simulink model "SIL_DCMotor"  (R2022b)
settings: Solver=VariableStepAuto  StartTime=0.0  StopTime=inf
values from neighbouring files (symbols this model uses):
  b = 0.1    [SIL_DCMotor_Parameter.m]
  J = 0.01    [SIL_DCMotor_Parameter.m]
  Kd_1 = 0.1    [SIL_DCMotor_Parameter.m]
  Kd_2 = 0.1    [SIL_DCMotor_Parameter.m]
  Ke = 0.367    [SIL_DCMotor_Parameter.m]
  Ki_1 = 0.1    [SIL_DCMotor_Parameter.m]
  Ki_2 = 0.75    [SIL_DCMotor_Parameter.m]
  Kp_1 = 0.5    [SIL_DCMotor_Parameter.m]
  Kp_2 = 7.5    [SIL_DCMotor_Parameter.m]
  Kt = 0.367    [SIL_DCMotor_Parameter.m]
  L = 0.5    [SIL_DCMotor_Parameter.m]
  R = 0.1    [SIL_DCMotor_Parameter.m]
  T_L = 0    [SIL_DCMotor_Parameter.m]
  T_sil = 1    [SIL_DCMotor_Parameter.m]
undefined symbols (not defined in the file or in its folder): LF
libraries: fl_lib x5, nesl_utility x4, ee_lib x3, instrumentseriallib x3, slpidlib x2, etargetslib x1
settings Model: Creator=Bramantio  LastModifiedBy=Bramantio

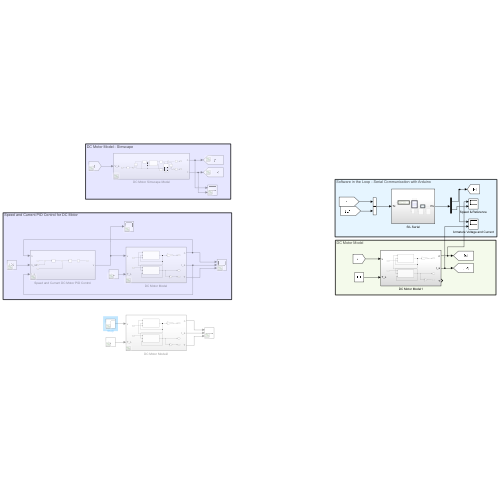
[thumbnail: Simulink's stored preview of the top-level diagram]
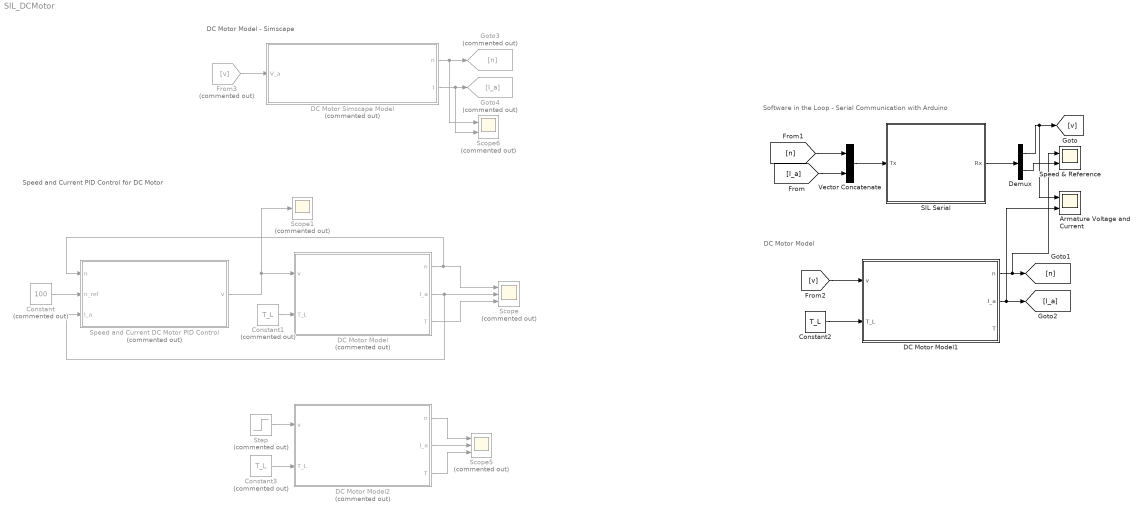
== system SIL_DCMotor ==
  note: DC Motor Model - Simscape
  note: DC Motor Model
  note: Speed and Current PID Control for DC Motor
  note: Software in the Loop - Serial Communication with Arduino
  Armature Voltage and Current : Scope  NumInputPorts=2
  Constant : Constant  Commented=on  Value=100
  Constant1 : Constant  Commented=on  Value=T_L
  Constant2 : Constant  Value=T_L
  Constant3 : Constant  Commented=on  Value=T_L
  DC Motor Model : Subsystem  Commented=on
  DC Motor Model1 : Subsystem
  DC Motor Model2 : Subsystem  Commented=on
  DC Motor Simscape Model : Subsystem  Commented=on
  Demux : Demux  Outputs=2
  From3 : From  Commented=on  GotoTag=v
  Goto3 : Goto  Commented=on  GotoTag=n
  Goto4 : Goto  Commented=on  GotoTag=I_a
  SIL Serial : Subsystem
  Scope : Scope  Commented=on  NumInputPorts=3
  Scope1 : Scope  Commented=on
  Scope5 : Scope  Commented=on  NumInputPorts=3
  Scope6 : Scope  Commented=on  NumInputPorts=2
  Speed & Reference : Scope  NumInputPorts=2
  Speed and Current DC Motor PID Control : Subsystem  Commented=on
  Step : Step  Commented=on  Time=5  After=12  SampleTime=0
  Vector Concatenate : Concatenate
  wires:
  SIL Serial/1(Rx) -> Demux/1
  Demux/2 -> Speed & Reference/2
  [n] -> Vector Concatenate/1
  Demux/1 -> Armature Voltage and Current/1, [v]
  [I_a] -> Vector Concatenate/2
  Vector Concatenate/1 -> SIL Serial/1(Tx)
  DC Motor Model/2(I_a) -> Scope/2, Speed and Current DC Motor PID Control/3(I_a)
  Constant1/1 -> DC Motor Model/2(T_L)
  Constant/1 -> Speed and Current DC Motor PID Control/2(n_ref)
  Speed and Current DC Motor PID Control/1(v) -> Scope1/1, DC Motor Model/1(v)
  DC Motor Model/3(T) -> Scope/3
  DC Motor Model/1(n) -> Scope/1, Speed and Current DC Motor PID Control/1(n)
  Constant2/1 -> DC Motor Model1/2(T_L)
  [v] -> DC Motor Model1/1(v)
  DC Motor Model1/2(I_a) -> Armature Voltage and Current/2, [I_a]
  Constant3/1 -> DC Motor Model2/2(T_L)
  Step/1 -> DC Motor Model2/1(v)
  DC Motor Model2/2(I_a) -> Scope5/2
  DC Motor Model2/1(n) -> Scope5/1
  DC Motor Model2/3(T) -> Scope5/3
  DC Motor Simscape Model/1(n) -> Scope6/1, Goto3/1
  From3/1 -> DC Motor Simscape Model/1(V_a)
  DC Motor Simscape Model/2(I) -> Scope6/2, Goto4/1
  DC Motor Model1/1(n) -> Speed & Reference/1, [n]

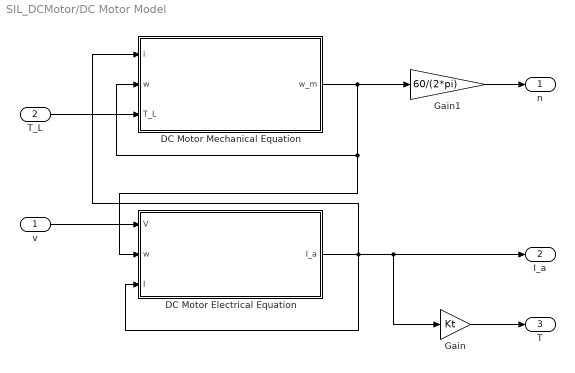
== system SIL_DCMotor/DC Motor Model ==
  v : Inport
  T_L : Inport  Port=2
  DC Motor Electrical Equation : Subsystem
  DC Motor Mechanical Equation : Subsystem
  Gain : Gain  Gain=Kt
  Gain1 : Gain  Gain=60/(2*pi)
  n : Outport
  I_a : Outport  Port=2
  T : Outport  Port=3
  wires:
  DC Motor Mechanical Equation/1(w_m) -> Gain1/1, DC Motor Electrical Equation/2(w), DC Motor Mechanical Equation/2(w)
  v/1 -> DC Motor Electrical Equation/1(V)
  Gain1/1 -> n/1
  DC Motor Electrical Equation/1(I_a) -> DC Motor Mechanical Equation/1(i), Gain/1, I_a/1, DC Motor Electrical Equation/3(I)
  Gain/1 -> T/1
  T_L/1 -> DC Motor Mechanical Equation/3(T_L)

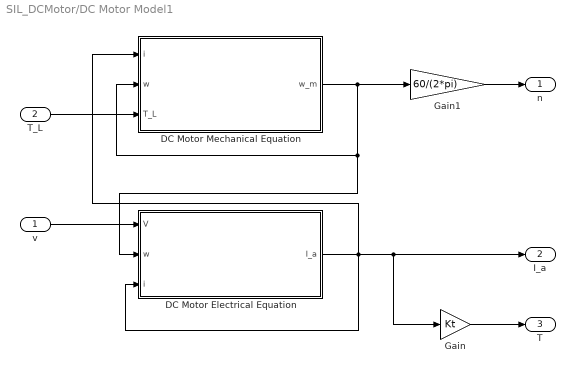
== system SIL_DCMotor/DC Motor Model1 ==
  v : Inport
  T_L : Inport  Port=2
  DC Motor Electrical Equation : Subsystem
  DC Motor Mechanical Equation : Subsystem
  Gain : Gain  Gain=Kt
  Gain1 : Gain  Gain=60/(2*pi)
  n : Outport
  I_a : Outport  Port=2
  T : Outport  Port=3
  wires:
  DC Motor Mechanical Equation/1(w_m) -> Gain1/1, DC Motor Electrical Equation/2(w), DC Motor Mechanical Equation/2(w)
  v/1 -> DC Motor Electrical Equation/1(V)
  Gain1/1 -> n/1
  DC Motor Electrical Equation/1(I_a) -> DC Motor Mechanical Equation/1(i), Gain/1, I_a/1, DC Motor Electrical Equation/3(i)
  Gain/1 -> T/1
  T_L/1 -> DC Motor Mechanical Equation/3(T_L)

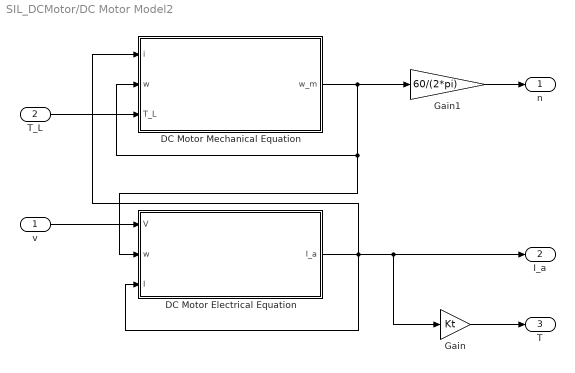
== system SIL_DCMotor/DC Motor Model2 ==
  v : Inport
  T_L : Inport  Port=2
  DC Motor Electrical Equation : Subsystem
  DC Motor Mechanical Equation : Subsystem
  Gain : Gain  Gain=Kt
  Gain1 : Gain  Gain=60/(2*pi)
  n : Outport
  I_a : Outport  Port=2
  T : Outport  Port=3
  wires:
  DC Motor Mechanical Equation/1(w_m) -> Gain1/1, DC Motor Electrical Equation/2(w), DC Motor Mechanical Equation/2(w)
  v/1 -> DC Motor Electrical Equation/1(V)
  Gain1/1 -> n/1
  DC Motor Electrical Equation/1(I_a) -> DC Motor Mechanical Equation/1(i), Gain/1, I_a/1, DC Motor Electrical Equation/3(I)
  Gain/1 -> T/1
  T_L/1 -> DC Motor Mechanical Equation/3(T_L)

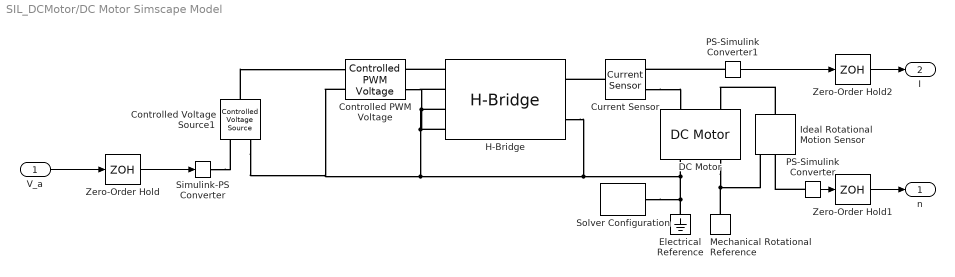
== system SIL_DCMotor/DC Motor Simscape Model ==
  V_a : Inport
  Controlled PWM Voltage : ee_lib/Integrated Circuits/Controlled PWM Voltage  F=4000 Hz  TD=0 s  pulse_width_offset=0 s  pulse_min=0 s  pwm_or_av=ee.enum.pwm_or_av.averaged  event_type=ee.enum.ic.event.asynchronous  sample_time=1e-6 s  Vmin=0 V  Vmax=5 V  Vm=5 V  u_min=0  u_max=1
  Controlled Voltage Source1 : fl_lib/Electrical/Electrical Sources/Controlled Voltage Source
  Current Sensor : fl_lib/Electrical/Electrical Sensors/Current Sensor
  DC Motor : ee_lib/Electromechanical/Brushed Motors/DC Motor  field_option=ee.enum.field_option.pm  Rf=100 Ohm  Lf=1 H  Laf=0.15 H  If0=0 A  parameterization=ee.enum.dcparam_option.circuit_param  Ra=R Ohm  La=L H  emf_or_torque=ee.enum.emf_or_torque.ki  Kv=Kt V/rpm  Ki=Ke N*m/A  T_stall=0.24e-3 N*m  w_max=4000 rpm  w_rated=2500 rpm  P_rated=10 W  V_rated=12 V  lam_param=ee.enum.lam_param.damping  i_noload=0 A  V_i_noload=1.5 V  J=J kg*m^2  lam=b N*m*s/rad  speed0=0 rpm  enable_fault_armature=simscape.enum.onoff.off  rev_faulted=1 / 3  G_faulted_armature=1e-5 S  fault_trigger_armature=ee.enum.faults.faultTrigger.temporal  t_fault_armature=1 s  max_permissible_current_armature=inf A  t_fail_on_current_armature=1 s  enable_fault_field=simscape.enum.onoff.off  G_faulted_field=1e-5 S  fault_trigger_field=ee.enum.faults.faultTrigger.temporal  t_fault_field=1 s  max_permissible_current_field=inf A  t_fail_on_current_field=1 s  fault_action=simscape.enum.assert.action.none  alpha=3.93e-3 1/K  Tmeas=25 degC  thermal_mass=100 J/K  initial_temperature=25 degC
  Electrical Reference : fl_lib/Electrical/Electrical Elements/Electrical Reference
  H-Bridge : ee_lib/Semiconductors & Converters/Converters/H-Bridge  supply_ports=ee.enum.supply_ports.hidesupply  pwm_or_av=ee.enum.pwm_or_av.averaged  regenerative_braking_mode=ee.enum.converters.regenerative_braking_mode.depends_on_rev  discontinuous=ee.enum.current_profile.continuous  freewheeling_mode=ee.enum.converters.freewheeling_mode.one_switch_one_diode  Rload=10 Ohm  Lload=1e-5 H  F=10 kHz  Venable=2.5 V  Vmax=5.0 V  Vreverse=2.5 V  Vbrake=2.5 V  Vm=12 V  Ron=0.1 Ohm  Don=0.05 Ohm  Goff=1e-6 S  Tmeas=298.15 K  Ron2=0.1 Ohm  Don2=0.05 Ohm  Tmeas2=398.15 K  thermal_mass=100 J/K  initial_temperature=298.15 K
  Ideal Rotational Motion Sensor : fl_lib/Mechanical/Mechanical Sensors/Ideal Rotational Motion Sensor  reference=foundation.enum.MeasurementReference.difference  acceleration_port=false  velocity_port=true  position_port=true  wrap_angle=false  offset=0 rad
  Mechanical Rotational Reference : fl_lib/Mechanical/Rotational Elements/Mechanical Rotational Reference
  PS-Simulink Converter : nesl_utility/PS-Simulink Converter  PhysicalDomain=network_engine_domain  SubClassName=ps_output  LeftPortType=input  RightPortType=output  PseudoPeriodic=off  Frequencies=[]  VectorFormat=inherit  Unit=rpm  AffineConversion=off
  PS-Simulink Converter1 : nesl_utility/PS-Simulink Converter  PhysicalDomain=network_engine_domain  SubClassName=ps_output  LeftPortType=input  RightPortType=output  PseudoPeriodic=off  Frequencies=[]  VectorFormat=inherit  Unit=A  AffineConversion=off
  Simulink-PS Converter : nesl_utility/Simulink-PS Converter  PhysicalDomain=network_engine_domain  SubClassName=ps_input  LeftPortType=input  RightPortType=output  PseudoPeriodic=off  Frequencies=[]  NoiseDistribution=none  NoiseParameters=[]  Unit=1  AffineConversion=off  FilteringAndDerivatives=provide  SimscapeFilterOrder=1  InputFilterTimeConstant=0.001  UdotUserProvided=0
  Solver Configuration : nesl_utility/Solver Configuration  PhysicalDomain=network_engine_domain  SubClassName=solver  LeftPortType=input  RightPortType=generic  Tones=[]  Harmonics=[]  SimulateNoise=off  Profile=off  UseLocalSampling=off  EnableSwitchedLinearOptims=on  FrequencyDomain=off  UseCCode=off  RelTol=0.001  AbsTol=0.001  MinStep=1e-09  ToWorkspace=off  RevertToSquareIcSolve=off  NumHomotopyIterations=100  PhasorMode=off  PhasorModeNumHarmonics=1  ConsistencySolver=NEWTON_XTOL_AFTER_FTOL  IndexReductionMethod=DerivativeReplacement  DoDC=off  ResidualTolerance=1e-09  ConsistencyTolSource=GLOBAL  ConsistencyAbsTol=0.001  ConsistencyRelTol=0.001  ConsistencyTolFactor=0.001  UseLocalSolver=off  LocalSolverChoice=NE_BACKWARD_EULER_ADVANCER  ResolveIndetEquations=on  FunctionEvalNumThread=1  LocalSolverSampleTime=0.001  DoFixedCost=off  MaxNonlinIter=3  MaxModeIter=2  ComputeImpulses=off  ImpulseIterations=2  LinearAlgebra=auto  LinearAlgebraNumThread=0  EquationFormulation=NE_TIME_EF  DelaysMemoryBudget=1024  AutomaticFiltering=on  FilteringTimeConstant=0.001  PartitionStorageMethod=AS_NEEDED  PartitionMemoryBudget=1024  PartitionMethod=ROBUST
  Zero-Order Hold : ZeroOrderHold  SampleTime=T_sil
  Zero-Order Hold1 : ZeroOrderHold  SampleTime=T_sil
  Zero-Order Hold2 : ZeroOrderHold  SampleTime=T_sil
  n : Outport
  I : Outport  Port=2
  wires:
  PS-Simulink Converter1/1 -> Zero-Order Hold2/1
  V_a/1 -> Zero-Order Hold/1
  Zero-Order Hold/1 -> Simulink-PS Converter/1
  PS-Simulink Converter/1 -> Zero-Order Hold1/1
  Zero-Order Hold1/1 -> n/1
  Zero-Order Hold2/1 -> I/1
  connections:
  Current Sensor/LConn1 -- H-Bridge/RConn1
  Electrical Reference/LConn1 -- Solver Configuration/RConn1 -- H-Bridge/RConn2 -- Controlled Voltage Source1/RConn2 -- Controlled PWM Voltage/LConn2 -- Controlled PWM Voltage/RConn2 -- H-Bridge/LConn2 -- H-Bridge/LConn3 -- H-Bridge/LConn4 -- DC Motor/RConn1
  Controlled Voltage Source1/LConn1 -- Controlled PWM Voltage/LConn1
  Current Sensor/RConn2 -- DC Motor/LConn1
  H-Bridge/LConn1 -- Controlled PWM Voltage/RConn1
  PS-Simulink Converter1/LConn1 -- Current Sensor/RConn1
  Mechanical Rotational Reference/LConn1 -- DC Motor/RConn2 -- Ideal Rotational Motion Sensor/RConn1
  PS-Simulink Converter/LConn1 -- Ideal Rotational Motion Sensor/RConn2
  Ideal Rotational Motion Sensor/LConn1 -- DC Motor/LConn2
  Simulink-PS Converter/RConn1 -- Controlled Voltage Source1/RConn1

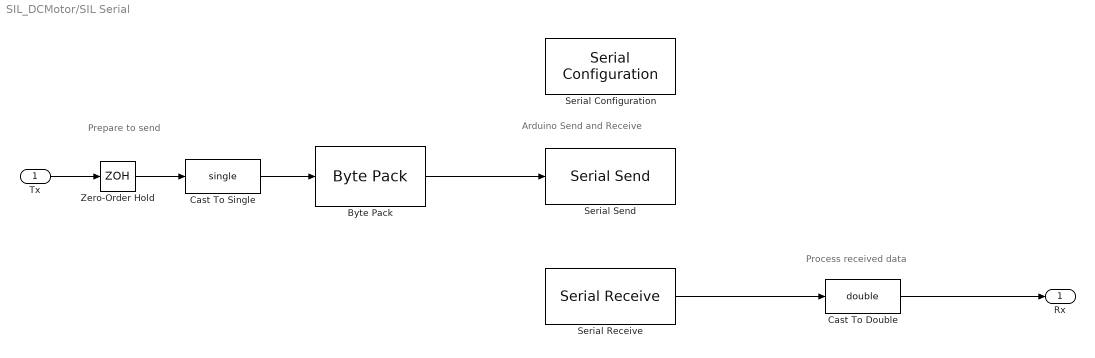
== system SIL_DCMotor/SIL Serial ==
  note: Prepare to send
  note: Arduino Send and Receive
  note: Process received data
  Tx : Inport
  Byte Pack : etargetslib/Byte Pack  datatypes={'single'}  byteAlign=4
  Cast To Double : DataTypeConversion  OutDataTypeStr=double  SaturateOnIntegerOverflow=off  RndMeth=Floor
  Cast To Single : DataTypeConversion  OutDataTypeStr=single  SaturateOnIntegerOverflow=off  RndMeth=Floor
  Serial Configuration : instrumentseriallib/Serial Configuration  Priority=-200000  PortSel=COM7  Port=COM7  ComPort=COM7  BaudRate=BaudRate  DataBits=8  Parity=none  StopBits=1  ByteOrder=little-endian  FlowControl=none  Timeout=10  SimulateUsing=Interpreted execution  BlockInModel=on  aMode=1
  Serial Receive : instrumentseriallib/Serial Receive  Priority=1  PortSel=COM7  Port=COM7  ComPort=COM7  DataType=single  SaveDataType=uint8  ToggleHeader=on  Header=[ 65 ]  ToggleTerminator=on  Terminator=LF ('\n')  CustomTerminator=[]  InputFormat=Column major  ToggleDataSize=on  DataSize=[1 2]  EnableBlockingMode=on  ActionDataUnavailable=Output last received value  ActionWhenDataUnavailable=Output last received value  CustomValue=0  SampleTime=T_sil  SimulateUsing=Interpreted execution  BlockInModel=on  aMode=1
  Serial Send : instrumentseriallib/Serial Send  Priority=1  PortSel=COM7  Port=COM7  ComPort=COM7  Header=[]  Terminator=LF ('\n')  CustomTerminator=[]  EnableBlockingMode=on  SimulateUsing=Interpreted execution  BlockInModel=on  aMode=1
  Zero-Order Hold : ZeroOrderHold  SampleTime=T_sil
  Rx : Outport
  wires:
  Tx/1 -> Zero-Order Hold/1
  Serial Receive/1 -> Cast To Double/1
  Zero-Order Hold/1 -> Cast To Single/1
  Byte Pack/1 -> Serial Send/1
  Cast To Double/1 -> Rx/1
  Cast To Single/1 -> Byte Pack/1

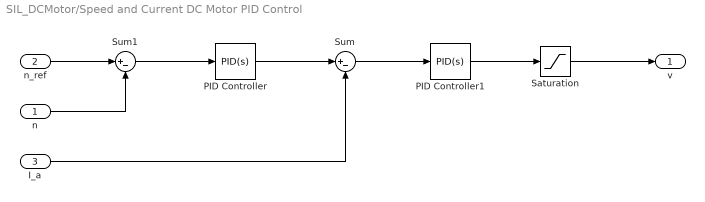
== system SIL_DCMotor/Speed and Current DC Motor PID Control ==
  n : Inport
  n_ref : Inport  Port=2
  I_a : Inport  Port=3
  PID Controller : slpidlib/PID Controller  Controller=PID  Form=Parallel  TimeDomain=Continuous-time  UseExternalTs=off  SampleTime=-1  IntegratorMethod=Forward Euler  FilterMethod=Forward Euler  ControllerParametersSource=internal  P=Kp_1  I=Ki_1  UseKiTs=off  D=Kd_1  N=13.8732743548756  UseFilter=on  TunerSelectOption=Transfer Function Based (PID Tuner App)  InitialConditionSource=internal  InitialConditionForIntegrator=0  InitialConditionForFilter=0  DifferentiatorICPrevScaledInput=0  ExternalReset=none  TrackingMode=off  Kt=1  LimitOutput=off  SatLimitsSource=internal  UpperSaturationLimit=inf  LowerSaturationLimit=-inf  LinearizeAsGain=on  AntiWindupMode=none  Kb=1  LimitIntegrator=off  UpperIntegratorSaturationLimit=inf  LowerIntegratorSaturationLimit=-inf  POutMin=[]  POutMax=[]  IOutMin=[]  IOutMax=[]  DOutMin=[]  DOutMax=[]  NOutMin=[]  NOutMax=[]  SumOutMin=[]  SumOutMax=[]  SaturationOutMin=[]  SaturationOutMax=[]  PParamMin=[]  PParamMax=[]  IParamMin=[]  IParamMax=[]  DParamMin=[]  DParamMax=[]  NParamMin=[]  NParamMax=[]  KbParamMin=[]  KbParamMax=[]  KtParamMin=[]  KtParamMax=[]  KbOutMin=[]  KbOutMax=[]  KtOutMin=[]  KtOutMax=[]  IntegratorOutMin=[]  IntegratorOutMax=[]  FilterOutMin=[]  FilterOutMax=[]  SumI1OutMin=[]  SumI1OutMax=[]  SumI2OutMin=[]  SumI2OutMax=[]  SumI3OutMin=[]  SumI3OutMax=[]  SumI4OutMin=[]  SumI4OutMax=[]  SumDOutMin=[]  SumDOutMax=[]  DifferentiatorOutMin=[]  DifferentiatorOutMax=[]  FilterDiffOutCoefMin=[]  FilterDiffOutCoefMax=[]  ReciprocalOutMin=[]  ReciprocalOutMax=[]  SumDenOutMin=[]  SumDenOutMax=[]  SumNumOutMin=[]  SumNumOutMax=[]  DivideOutMin=[]  DivideOutMax=[]  UdiffTsProdOutMin=[]  UdiffTsProdOutMax=[]  NTsProdOutMin=[]  NTsProdOutMax=[]  UintegralTsProdOutMin=[]  UintegralTsProdOutMax=[]  UngainTsProdOutMin=[]  UngainTsProdOutMax=[]  ClampingZeroOutDataTypeStr=Inherit: Inherit via back propagation  ClampingZeroOutMin=[]  ClampingZeroOutMax=[]  FilterDenConstantOutDataTypeStr=Inherit: Inherit via back propagation  FilterDenConstantOutMin=[]  FilterDenConstantOutMax=[]  PCopyOutDataTypeStr=Inherit: Inherit via back propagation  PCopyOutMin=[]  PCopyOutMax=[]  NCopyOutDataTypeStr=Inherit: Inherit via back propagation  NCopyOutMin=[]  NCopyOutMax=[]  IntegratorContinuousStateAttributes=''  IntegratorStateMustResolveToSignalObject=off  IntegratorRTWStateStorageClass=Auto  FilterContinuousStateAttributes=''  FilterStateMustResolveToSignalObject=off  FilterRTWStateStorageClass=Auto  ParallelPVariant=InternalParameters  IdealPVariant=Disabled  IVariant=InternalParameters  DVariant=InternalParameters  IntegratorVariant=Continuous  SatVariant=Disabled  AWVariant=Passthrough  PCopyVariant=Disabled  TRVariant=Disabled  FdbkBlocksVariant=Forward  IdealPFdbkVariant=Disabled  SatFdbkVariant=Disabled  DerivativeFilterVariant=ContFilter  NVariant=InternalParameters  NCopyVariant=Disabled  FilterICVariant=InternalICsFilter  IntegratorICVariant=InternalICs  ExternalResetVariant=Disabled  TRSumVariant=Passthrough  SumFdbkVariant=Disabled  SumVariant=Sum_PID  TsampFilterVariant=InternalTs  TsampNgainVariant=Passthrough  TsampIntegralVariant=Passthrough  ExternalSaturationOutDataTypeStr=Inherit: Same as second input
  PID Controller1 : slpidlib/PID Controller  Controller=PID  Form=Parallel  TimeDomain=Continuous-time  UseExternalTs=off  SampleTime=-1  IntegratorMethod=Forward Euler  FilterMethod=Forward Euler  ControllerParametersSource=internal  P=Kp_2  I=Ki_2  UseKiTs=off  D=Kd_2  N=100  UseFilter=on  TunerSelectOption=Transfer Function Based (PID Tuner App)  InitialConditionSource=internal  InitialConditionForIntegrator=0  InitialConditionForFilter=0  DifferentiatorICPrevScaledInput=0  ExternalReset=none  TrackingMode=off  Kt=1  LimitOutput=off  SatLimitsSource=internal  UpperSaturationLimit=inf  LowerSaturationLimit=-inf  LinearizeAsGain=on  AntiWindupMode=none  Kb=1  LimitIntegrator=off  UpperIntegratorSaturationLimit=inf  LowerIntegratorSaturationLimit=-inf  POutMin=[]  POutMax=[]  IOutMin=[]  IOutMax=[]  DOutMin=[]  DOutMax=[]  NOutMin=[]  NOutMax=[]  SumOutMin=[]  SumOutMax=[]  SaturationOutMin=[]  SaturationOutMax=[]  PParamMin=[]  PParamMax=[]  IParamMin=[]  IParamMax=[]  DParamMin=[]  DParamMax=[]  NParamMin=[]  NParamMax=[]  KbParamMin=[]  KbParamMax=[]  KtParamMin=[]  KtParamMax=[]  KbOutMin=[]  KbOutMax=[]  KtOutMin=[]  KtOutMax=[]  IntegratorOutMin=[]  IntegratorOutMax=[]  FilterOutMin=[]  FilterOutMax=[]  SumI1OutMin=[]  SumI1OutMax=[]  SumI2OutMin=[]  SumI2OutMax=[]  SumI3OutMin=[]  SumI3OutMax=[]  SumI4OutMin=[]  SumI4OutMax=[]  SumDOutMin=[]  SumDOutMax=[]  DifferentiatorOutMin=[]  DifferentiatorOutMax=[]  FilterDiffOutCoefMin=[]  FilterDiffOutCoefMax=[]  ReciprocalOutMin=[]  ReciprocalOutMax=[]  SumDenOutMin=[]  SumDenOutMax=[]  SumNumOutMin=[]  SumNumOutMax=[]  DivideOutMin=[]  DivideOutMax=[]  UdiffTsProdOutMin=[]  UdiffTsProdOutMax=[]  NTsProdOutMin=[]  NTsProdOutMax=[]  UintegralTsProdOutMin=[]  UintegralTsProdOutMax=[]  UngainTsProdOutMin=[]  UngainTsProdOutMax=[]  ClampingZeroOutDataTypeStr=Inherit: Inherit via back propagation  ClampingZeroOutMin=[]  ClampingZeroOutMax=[]  FilterDenConstantOutDataTypeStr=Inherit: Inherit via back propagation  FilterDenConstantOutMin=[]  FilterDenConstantOutMax=[]  PCopyOutDataTypeStr=Inherit: Inherit via back propagation  PCopyOutMin=[]  PCopyOutMax=[]  NCopyOutDataTypeStr=Inherit: Inherit via back propagation  NCopyOutMin=[]  NCopyOutMax=[]  IntegratorContinuousStateAttributes=''  IntegratorStateMustResolveToSignalObject=off  IntegratorRTWStateStorageClass=Auto  FilterContinuousStateAttributes=''  FilterStateMustResolveToSignalObject=off  FilterRTWStateStorageClass=Auto  ParallelPVariant=InternalParameters  IdealPVariant=Disabled  IVariant=InternalParameters  DVariant=InternalParameters  IntegratorVariant=Continuous  SatVariant=Disabled  AWVariant=Passthrough  PCopyVariant=Disabled  TRVariant=Disabled  FdbkBlocksVariant=Forward  IdealPFdbkVariant=Disabled  SatFdbkVariant=Disabled  DerivativeFilterVariant=ContFilter  NVariant=InternalParameters  NCopyVariant=Disabled  FilterICVariant=InternalICsFilter  IntegratorICVariant=InternalICs  ExternalResetVariant=Disabled  TRSumVariant=Passthrough  SumFdbkVariant=Disabled  SumVariant=Sum_PID  TsampFilterVariant=InternalTs  TsampNgainVariant=Passthrough  TsampIntegralVariant=Passthrough  ExternalSaturationOutDataTypeStr=Inherit: Same as second input
  Saturation : Saturate  UpperLimit=12  LowerLimit=0
  Sum : Sum  Inputs=|+-
  Sum1 : Sum  Inputs=|+-
  v : Outport
  wires:
  n_ref/1 -> Sum1/1
  I_a/1 -> Sum/2
  Sum1/1 -> PID Controller/1
  Sum/1 -> PID Controller1/1
  n/1 -> Sum1/2
  PID Controller1/1 -> Saturation/1
  Saturation/1 -> v/1
  PID Controller/1 -> Sum/1

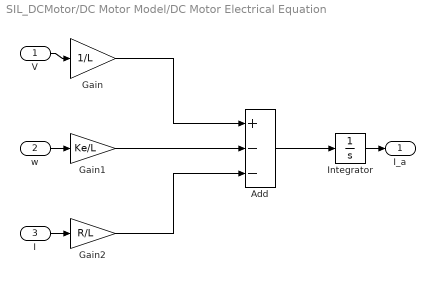
== system SIL_DCMotor/DC Motor Model/DC Motor Electrical Equation ==
  V : Inport
  w : Inport  Port=2
  I : Inport  Port=3
  Add : Sum  Inputs=+--
  Gain : Gain  Gain=1/L
  Gain1 : Gain  Gain=Ke/L
  Gain2 : Gain  Gain=R/L
  Integrator : Integrator
  I_a : Outport
  wires:
  V/1 -> Gain/1
  Gain2/1 -> Add/3
  Gain1/1 -> Add/2
  Add/1 -> Integrator/1
  I/1 -> Gain2/1
  Gain/1 -> Add/1
  Integrator/1 -> I_a/1
  w/1 -> Gain1/1

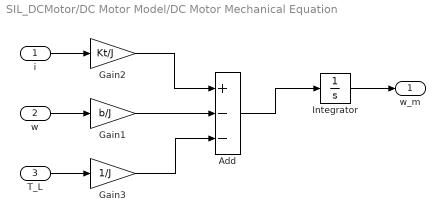
== system SIL_DCMotor/DC Motor Model/DC Motor Mechanical Equation ==
  i : Inport
  w : Inport  Port=2
  T_L : Inport  Port=3
  Add : Sum  Inputs=+--
  Gain1 : Gain  Gain=b/J
  Gain2 : Gain  Gain=Kt/J
  Gain3 : Gain  Gain=1/J
  Integrator : Integrator
  w_m : Outport
  wires:
  Add/1 -> Integrator/1
  i/1 -> Gain2/1
  Gain1/1 -> Add/2
  Integrator/1 -> w_m/1
  w/1 -> Gain1/1
  Gain2/1 -> Add/1
  Gain3/1 -> Add/3
  T_L/1 -> Gain3/1

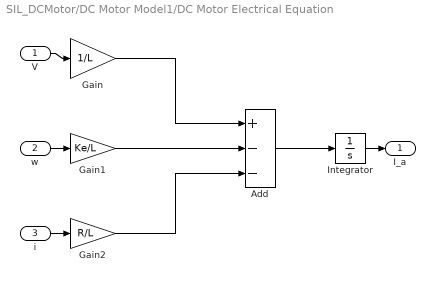
== system SIL_DCMotor/DC Motor Model1/DC Motor Electrical Equation ==
  V : Inport
  w : Inport  Port=2
  i : Inport  Port=3
  Add : Sum  Inputs=+--
  Gain : Gain  Gain=1/L
  Gain1 : Gain  Gain=Ke/L
  Gain2 : Gain  Gain=R/L
  Integrator : Integrator
  I_a : Outport
  wires:
  V/1 -> Gain/1
  Gain2/1 -> Add/3
  Gain1/1 -> Add/2
  Add/1 -> Integrator/1
  i/1 -> Gain2/1
  Gain/1 -> Add/1
  Integrator/1 -> I_a/1
  w/1 -> Gain1/1

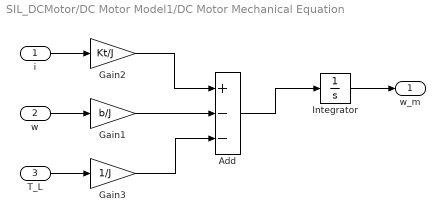
== system SIL_DCMotor/DC Motor Model1/DC Motor Mechanical Equation ==
  i : Inport
  w : Inport  Port=2
  T_L : Inport  Port=3
  Add : Sum  Inputs=+--
  Gain1 : Gain  Gain=b/J
  Gain2 : Gain  Gain=Kt/J
  Gain3 : Gain  Gain=1/J
  Integrator : Integrator
  w_m : Outport
  wires:
  Add/1 -> Integrator/1
  i/1 -> Gain2/1
  Gain1/1 -> Add/2
  Integrator/1 -> w_m/1
  w/1 -> Gain1/1
  Gain2/1 -> Add/1
  Gain3/1 -> Add/3
  T_L/1 -> Gain3/1

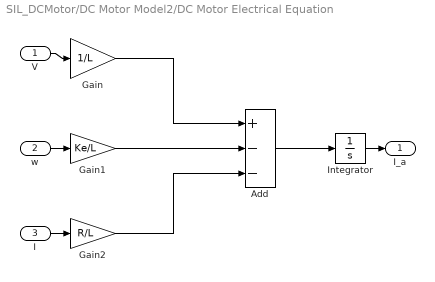
== system SIL_DCMotor/DC Motor Model2/DC Motor Electrical Equation ==
  V : Inport
  w : Inport  Port=2
  I : Inport  Port=3
  Add : Sum  Inputs=+--
  Gain : Gain  Gain=1/L
  Gain1 : Gain  Gain=Ke/L
  Gain2 : Gain  Gain=R/L
  Integrator : Integrator
  I_a : Outport
  wires:
  V/1 -> Gain/1
  Gain2/1 -> Add/3
  Gain1/1 -> Add/2
  Add/1 -> Integrator/1
  I/1 -> Gain2/1
  Gain/1 -> Add/1
  Integrator/1 -> I_a/1
  w/1 -> Gain1/1

== system SIL_DCMotor/DC Motor Model2/DC Motor Mechanical Equation ==
  i : Inport
  w : Inport  Port=2
  T_L : Inport  Port=3
  Add : Sum  Inputs=+--
  Gain1 : Gain  Gain=b/J
  Gain2 : Gain  Gain=Kt/J
  Gain3 : Gain  Gain=1/J
  Integrator : Integrator
  w_m : Outport
  wires:
  Add/1 -> Integrator/1
  i/1 -> Gain2/1
  Gain1/1 -> Add/2
  Integrator/1 -> w_m/1
  w/1 -> Gain1/1
  Gain2/1 -> Add/1
  Gain3/1 -> Add/3
  T_L/1 -> Gain3/1
